simulink subsystem "EvitarObstaculos"  (R2023b)
settings: Solver=VariableStepAuto  StartTime=0.0  StopTime=10.0  RelTol=1e-3
settings Model: Creator=pablo  LastModifiedBy=pablo

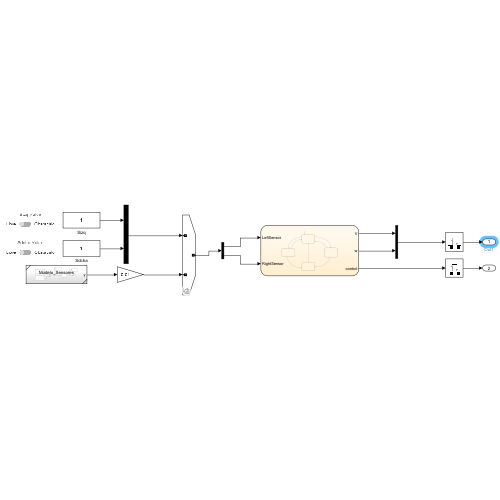
[thumbnail: Simulink's stored preview of the top-level diagram]
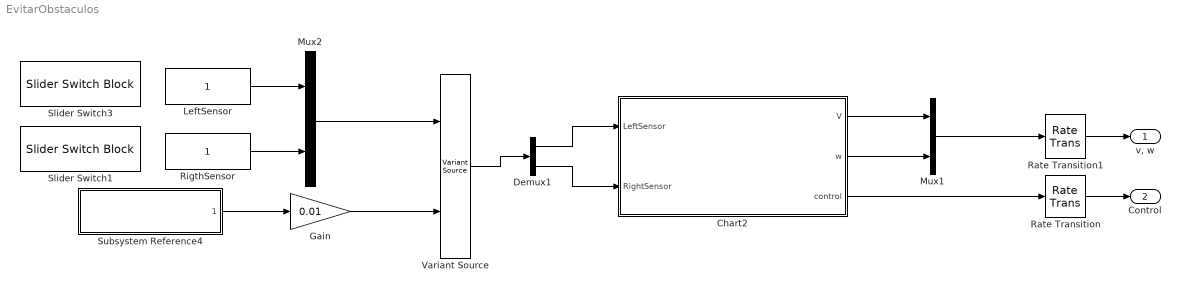
== system EvitarObstaculos ==
  Chart2 : Stateflow chart  TreatAsAtomicUnit=on
  Demux1 : Demux  Outputs=2
  Gain : Gain  Gain=0.01  OutDataTypeStr=double
  LeftSensor : Constant
  Mux1 : Mux  Inputs=2
  Mux2 : Mux  Inputs=2
  Rate Transition : RateTransition
  Rate Transition1 : RateTransition
  RigthSensor : Constant
  Slider Switch1 : SliderSwitchBlock
      settings: Values={{'Libre', 'Obstaculo'}, [1 0.29]}
  Slider Switch3 : SliderSwitchBlock
      settings: Values={{'Libre', 'Obstaculo'}, [1 0.29]}
  Subsystem Reference4 : Subsystem  ReferencedSubsystem=Modelo_Sensores
  Variant Source : VariantSource  VariantControlMode=sim codegen switching
  "v, w" : Outport
  Control : Outport  Port=2
  wires:
  Chart2/1(V) -> Mux1/1
  Mux1/1 -> Rate Transition1/1
  Chart2/3(control) -> Rate Transition/1
  Gain/1 -> Variant Source/2
  RigthSensor/1 -> Mux2/2
  Mux2/1 -> Variant Source/1
  LeftSensor/1 -> Mux2/1
  Subsystem Reference4/1 -> Gain/1
  Demux1/1 -> Chart2/1(LeftSensor)
  Variant Source/1 -> Demux1/1
  Demux1/2 -> Chart2/2(RightSensor)
  Rate Transition1/1 -> "v, w"/1
  Rate Transition/1 -> Control/1
  Chart2/2(w) -> Mux1/2

== stateflow chart EvitarObstaculos/Chart2 ==
  state SinObstaculos
    en:
    control = 0;
    V = 0.205;
    w = 0;
  state RecuperarOrioentacion1
    en:
    control = 1;
    V = 0.1;
    w = 1.4;
  state ObstaculoDcha
    en:
    control = 1;
    V = 0.1;
    w = 1.4;
  state ObstaculoIzq
    en:
    control = 1;
    V = 0.1;
    w = -1.4;
  state RecuperarOrioentacion2
    en:
    control = 1;
    V = 0.1;
    w = -1.4;
  state ObstaculoFrente
    en:
    control = 1;
    V = 0;
    w = 2.4;
  (default) -> SinObstaculos
  RecuperarOrioentacion2 -> SinObstaculos [order 1] : after(2,sec)
  RecuperarOrioentacion1 -> SinObstaculos [order 1] : after(2,sec)
  SinObstaculos -> ObstaculoDcha [order 2] : [RightSensor<0.3]
  SinObstaculos -> ObstaculoIzq [order 1] : [LeftSensor<0.3]
  ObstaculoFrente -> SinObstaculos : after(1,sec)
  ObstaculoDcha -> RecuperarOrioentacion2 [order 1] : after(1,sec)
  RecuperarOrioentacion1 -> ObstaculoIzq [order 2] : [LeftSensor<0.3]
  ObstaculoIzq -> RecuperarOrioentacion1 [order 1] : after(1,sec)
  RecuperarOrioentacion2 -> ObstaculoDcha [order 2] : [RightSensor<0.3]
  ObstaculoIzq -> ObstaculoFrente [order 2] : [RightSensor<0.3]
  ObstaculoDcha -> ObstaculoFrente [order 2] : [LeftSensor<0.3]
  data: V output double size=1; w output double size=1; LeftSensor input size=1; RightSensor input size=1; control output uint8 size=1
  data V settings: description=Velocidad lineal del vehiculo
